simulink subsystem "th11_Suspension"  (R2026a)
settings: Solver=VariableStepAuto
undefined symbols (not defined in the file): Chassis, Init
settings Model: Creator=th12-dv  LastModifiedBy=th12-dv

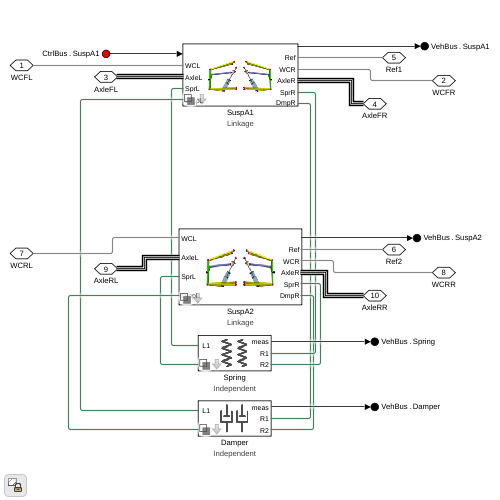
[thumbnail: Simulink's stored preview of the top-level diagram]
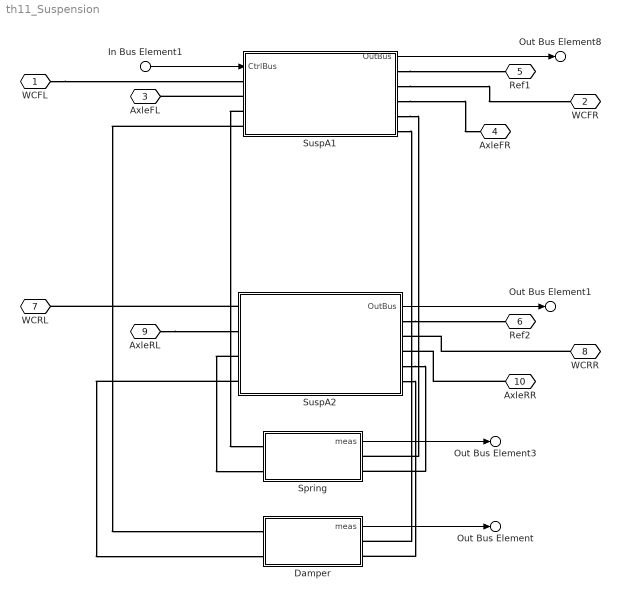
== system th11_Suspension ==
  In Bus Element1 : Inport  PortName=CtrlBus  Element=SuspA1
  Damper : Subsystem  Tag=PublishSubsystem  Variant=on  VariantControlMode=label  VariantControl=Variant1  LabelModeActiveChoice=Independent  mask(Variants for Dampers){Damper=Chassis.Damper, VariantLabel=Chassis.Damper.class.Value}
      mask prompts: Damper "Damper Parameters"; VariantLabel "Variant Label"
      mask help: Select option and provide parameters for left and right dampers on two axles. Option is chosen by string provided in Variant Label. The parameters for the selected option is contained in Dampers data structure.
      mask init:
      | curblk = gcb;
      | 
      | % Set variant for this block 
      | set_param(curblk,'LabelModeActiveChoice',VariantLabel);
      settings: AttributesFormatString=%<ActiveVariant>
      mask Display:
      | if(strcmp(get_param(gcb,'LabelModeActiveChoice'),'None'))
      |     disp(' ');
      | else
      |     image('sm_car_vehicle_chassis_damper_IMAGE.png');
      | end
  Spring : Subsystem  Tag=PublishSubsystem  Variant=on  VariantControlMode=label  VariantControl=Variant1  LabelModeActiveChoice=Independent  mask(Variants for Springs){Spring=Chassis.Spring, VariantLabel=Chassis.Spring.class.Value}
      mask prompts: Spring "Spring Parameters"; VariantLabel "Variant Label"
      mask help: Select option and provide parameters for left and right springs on two axles. Option is chosen by string provided in Variant Label. The parameters for the selected option is contained in Springs data structure.
      mask init:
      | curblk = gcb;
      | 
      | % Set variant for this block 
      | set_param(curblk,'LabelModeActiveChoice',VariantLabel);
      settings: AttributesFormatString=%<ActiveVariant>
      mask Display:
      | if(strcmp(get_param(gcb,'LabelModeActiveChoice'),'None'))
      |     disp(' ');
      | else
      |     image('sm_car_vehicle_chassis_spring_IMAGE.png');
      | end
  SuspA1 : Subsystem  Variant=on  VariantControlMode=label  VariantControl=Variant1  LabelModeActiveChoice=Linkage  mask(Suspension and Steering){Susp=Chassis.SuspA1, Init=Init.Axle1, VariantLabel=Chassis.SuspA1.class.Value}
      mask prompts: Susp "Suspension Parameters"; Init "Initial Values"; VariantLabel "Variant Label"
      mask help: Models suspension and optional steering system for one axle. Option is chosen by string provided in Variant Label. The parameters for the selected option are contained in Suspension Parameters data structure.
      mask init:
      | curblk = gcb;
      | 
      | % Set variant for this block 
      | set_param(curblk,'LabelModeActiveChoice',VariantLabel);
      settings: AttributesFormatString=%<LabelModeActiveChoice>
  SuspA2 : Subsystem  Variant=on  VariantControlMode=label  VariantControl=Variant1  LabelModeActiveChoice=Linkage  mask(Suspension and Steering){Susp=Chassis.SuspA2, Init=Init.Axle2, VariantLabel=Chassis.SuspA2.class.Value}
      mask prompts: Susp "Suspension Parameters"; Init "Initial Values"; VariantLabel "Variant Label"
      mask help: Models suspension and optional steering system for one axle. Option is chosen by string provided in Variant Label. The parameters for the selected option are contained in Suspension Parameters data structure.
      mask init:
      | curblk = gcb;
      | 
      | % Set variant for this block 
      | set_param(curblk,'LabelModeActiveChoice',VariantLabel);
      settings: AttributesFormatString=%<LabelModeActiveChoice>
  WCFL : PMIOPort  Side=Left
  WCFR : PMIOPort  Port=2  Side=Right
  AxleFL : PMIOPort  Port=3  Side=Left
  AxleFR : PMIOPort  Port=4  Side=Right
  Ref1 : PMIOPort  Port=5  Side=Right
  Ref2 : PMIOPort  Port=6  Side=Right
  WCRL : PMIOPort  Port=7  Side=Left
  WCRR : PMIOPort  Port=8  Side=Right
  AxleRL : PMIOPort  Port=9  Side=Left
  AxleRR : PMIOPort  Port=10  Side=Right
  Out Bus Element3 : Outport  VectorParamsAs1DForOutWhenUnconnected=off  PortName=VehBus  Element=Spring
  Out Bus Element8 : Outport  VectorParamsAs1DForOutWhenUnconnected=off  PortName=VehBus  Element=SuspA1
  Out Bus Element1 : Outport  VectorParamsAs1DForOutWhenUnconnected=off  PortName=VehBus  Element=SuspA2
  Out Bus Element : Outport  VectorParamsAs1DForOutWhenUnconnected=off  PortName=VehBus  Element=Damper
  wires:
  Damper/1(" meas") -> Out Bus Element/1
  Spring/1(" meas") -> Out Bus Element3/1
  SuspA1/1(OutBus) -> Out Bus Element8/1
  SuspA2/1(OutBus) -> Out Bus Element1/1
  In Bus Element1/1 -> SuspA1/1("CtrlBus ")
  connections:
  WCFL/RConn1 -- SuspA1/LConn1
  SuspA1/RConn5 -- Damper/RConn1
  SuspA2/RConn4 -- Spring/RConn2
  SuspA1/RConn4 -- Spring/RConn1
  SuspA1/LConn2 -- AxleFL/RConn1
  SuspA2/LConn3 -- Spring/LConn2
  SuspA1/LConn3 -- Spring/LConn1
  SuspA2/RConn5 -- Damper/RConn2
  SuspA1/LConn4 -- Damper/LConn1
  SuspA2/LConn4 -- Damper/LConn2
  SuspA2/LConn1 -- WCRL/RConn1
  AxleRL/RConn1 -- SuspA2/LConn2
  SuspA1/RConn1 -- Ref1/RConn1
  SuspA2/RConn1 -- Ref2/RConn1
  AxleRR/RConn1 -- SuspA2/RConn3
  WCRR/RConn1 -- SuspA2/RConn2
  SuspA1/RConn3 -- AxleFR/RConn1
  SuspA1/RConn2 -- WCFR/RConn1

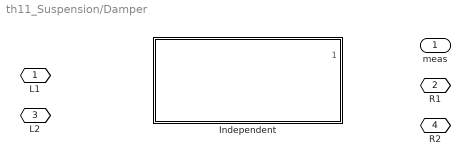
== system th11_Suspension/Damper ==
  Independent : Subsystem  VariantControl=Independent  ReferencedSubsystem=th11_Damper_Independent
  " L1" : PMIOPort  Side=Left
  " R1" : PMIOPort  Port=2  Side=Right
  " L2" : PMIOPort  Port=3  Side=Left
  " R2" : PMIOPort  Port=4  Side=Right
  " meas" : Outport  VectorParamsAs1DForOutWhenUnconnected=off

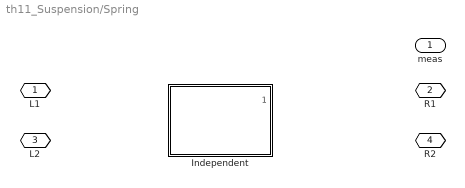
== system th11_Suspension/Spring ==
  Independent : Subsystem  VariantControl=Independent  ReferencedSubsystem=th11_Spring_Independent
  " L1" : PMIOPort  Side=Left
  R1 : PMIOPort  Port=2  Side=Right
  " L2" : PMIOPort  Port=3  Side=Left
  R2 : PMIOPort  Port=4  Side=Right
  " meas" : Outport  VectorParamsAs1DForOutWhenUnconnected=off

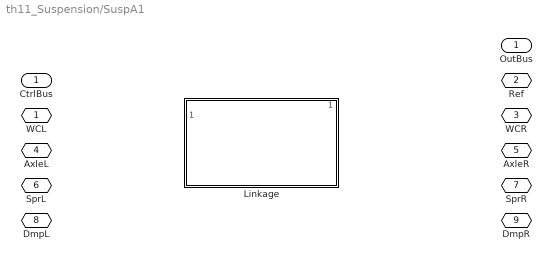
== system th11_Suspension/SuspA1 ==
  "CtrlBus " : Inport
  Linkage : Subsystem  VariantControl=Linkage  ReferencedSubsystem=th11_SuspA1_Linkage
  WCL : PMIOPort  Side=Left
  Ref : PMIOPort  Port=2  Side=Right
  WCR : PMIOPort  Port=3  Side=Right
  AxleL : PMIOPort  Port=4  Side=Left
  AxleR : PMIOPort  Port=5  Side=Right
  SprL : PMIOPort  Port=6  Side=Left
  SprR : PMIOPort  Port=7  Side=Right
  DmpL : PMIOPort  Port=8  Side=Left
  DmpR : PMIOPort  Port=9  Side=Right
  OutBus : Outport  VectorParamsAs1DForOutWhenUnconnected=off

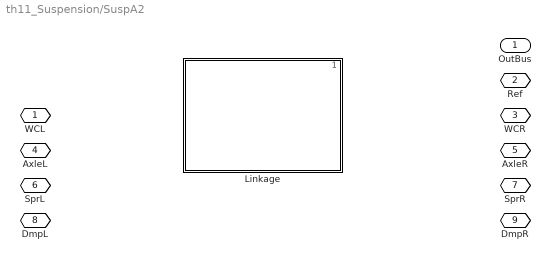
== system th11_Suspension/SuspA2 ==
  Linkage : Subsystem  VariantControl=Linkage  ReferencedSubsystem=th11_SuspA2_Linkage
  WCL : PMIOPort  Side=Left
  Ref : PMIOPort  Port=2  Side=Right
  WCR : PMIOPort  Port=3  Side=Right
  AxleL : PMIOPort  Port=4  Side=Left
  AxleR : PMIOPort  Port=5  Side=Right
  SprL : PMIOPort  Port=6  Side=Left
  SprR : PMIOPort  Port=7  Side=Right
  DmpL : PMIOPort  Port=8  Side=Left
  DmpR : PMIOPort  Port=9  Side=Right
  OutBus : Outport  VectorParamsAs1DForOutWhenUnconnected=off
